simulink model "FOC_physical_2"  (R2024b)
settings: Solver=FixedStepAuto  StartTime=0.0  StopTime=1  FixedStep=1e-6  RelTol=1e-3
undefined symbols (not defined in the file): alpha, DiscIntNeverNeededParam, Down, dspblkCoreblockFVToolHelper, gcbh, GPTRIP1SEL, Ki_current, Ki_q, Ki_s, Ki_speed, Kp_current, Kp_q, Kp_s, Kp_speed, lambda, lamdaM, Ld, Ls, ma, P, Rs, T_max, T_period, TZ1, Up, Vdc
libraries: c2802xlib x7, simulink x7, spsIGBTDiodeLib x6, spsCurrentMeasurementLib x3, eeStairGenerator x2, spsDCVoltageSourceLib x1, spsPermanentMagnetSynchronousMachineLib x1, mcbpositiondecoderlib x1, c281xlib x1, c280xlib x1, spspowerguiLib x1
(part 2 of 2)

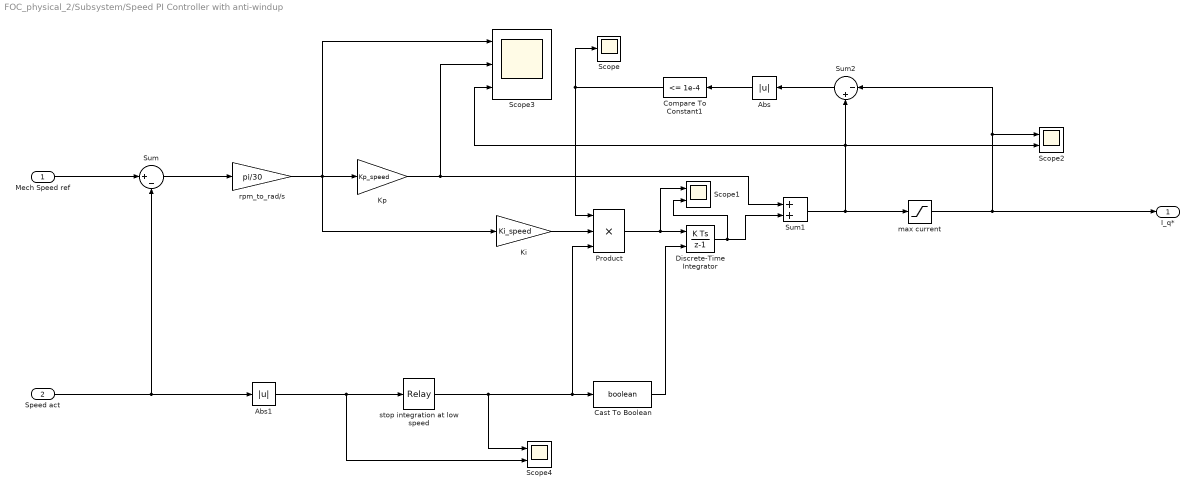
== system FOC_physical_2/Subsystem/Speed PI Controller with anti-windup ==
  Mech Speed ref : Inport
  Speed act : Inport  Port=2
  " max current" : Saturate  UpperLimit=T_max/((3/2)*lamdaM*P)  LowerLimit=0
  Abs : Abs  SaturateOnIntegerOverflow=off
  Abs1 : Abs  SaturateOnIntegerOverflow=off
  Cast To Boolean : DataTypeConversion  OutDataTypeStr=boolean  SaturateOnIntegerOverflow=off  RndMeth=Floor
  Compare To Constant1 : simulink/Logic and Bit Operations/Compare To Constant  relop=<=  const=1e-4  OutDataTypeStr=boolean
  Discrete-Time Integrator : DiscreteIntegrator  ExternalReset=falling  SampleTime=-1  ICPrevOutput=DiscIntNeverNeededParam  ICPrevScaledInput=DiscIntNeverNeededParam
  "Ki " : Gain  Gain=Ki_speed
  Kp : Gain  Gain=Kp_speed
  Product : Product  Inputs=3
  Scope : Scope
  Scope1 : Scope  NumInputPorts=2
  Scope2 : Scope  NumInputPorts=2
  Scope3 : Scope  NumInputPorts=3
  Scope4 : Scope  NumInputPorts=2
  Sum : Sum  Inputs=|+-
  Sum1 : Sum
  Sum2 : Sum  Inputs=|-+
  rpm_to_rad/s : Gain  Gain=pi/30
  stop integration at low speed : Relay  OnSwitchValue=100  OffSwitchValue=-100
  I_q* : Outport
  wires:
  " max current"/1 -> Scope2/1, Sum2/1, I_q*/1
  Sum/1 -> rpm_to_rad/s/1
  rpm_to_rad/s/1 -> Kp/1, Scope3/1, "Ki "/1
  stop integration at low speed/1 -> Cast To Boolean/1, Product/3, Scope4/1
  Abs1/1 -> Scope4/2, stop integration at low speed/1
  Compare To Constant1/1 -> Scope/1, Product/1
  Abs/1 -> Compare To Constant1/1
  Sum2/1 -> Abs/1
  Sum1/1 -> " max current"/1, Sum2/2, Scope3/3, Scope2/2
  Discrete-Time Integrator/1 -> Sum1/2, Scope1/2
  Product/1 -> Discrete-Time Integrator/1, Scope1/1
  "Ki "/1 -> Product/2
  Kp/1 -> Sum1/1, Scope3/2
  Speed act/1 -> Sum/2, Abs1/1
  Mech Speed ref/1 -> Sum/1
  Cast To Boolean/1 -> Discrete-Time Integrator/2

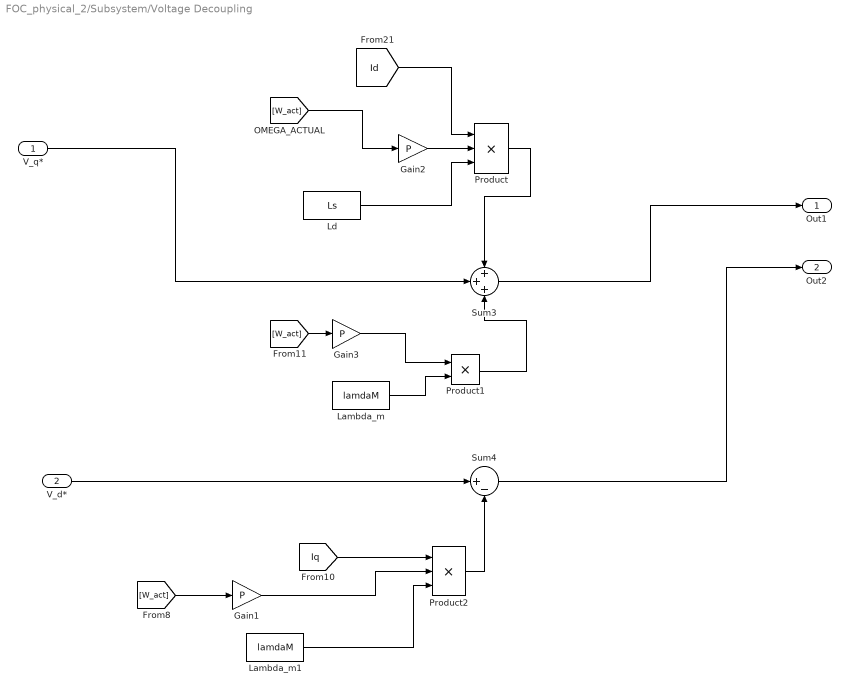
== system FOC_physical_2/Subsystem/Voltage Decoupling  ==
  V_q* : Inport
  V_d* : Inport  Port=2
  Gain1 : Gain  Gain=P
  Gain2 : Gain  Gain=P
  Gain3 : Gain  Gain=P
  Lambda_m : Constant  Value=lamdaM
  Lambda_m1 : Constant  Value=lamdaM
  Ld : Constant  Value=Ls
  Product : Product  Inputs=3
  Product1 : Product
  Product2 : Product  Inputs=3
  Sum3 : Sum  Inputs=+++
  Sum4 : Sum  Inputs=|+-
  Out1 : Outport
  Out2 : Outport  Port=2
  wires:
  [Id] -> Product/1
  V_q*/1 -> Sum3/2
  Gain1/1 -> Product2/2
  Product2/1 -> Sum4/2
  [Iq] -> Product2/1
  Product1/1 -> Sum3/3
  [W_act] -> Gain1/1
  Gain2/1 -> Product/2
  [W_act] -> Gain2/1
  Ld/1 -> Product/3
  [W_act] -> Gain3/1
  Product/1 -> Sum3/1
  Gain3/1 -> Product1/1
  Lambda_m/1 -> Product1/2
  Lambda_m1/1 -> Product2/3
  Sum3/1 -> Out1/1
  V_d*/1 -> Sum4/1
  Sum4/1 -> Out2/1

== system FOC_physical_2/Subsystem/d-current PI controller with anti-windup ==
  Id command : Inport
  Id act : Inport  Port=2
  Discrete-Time Integrator : DiscreteIntegrator  SampleTime=-1  ICPrevOutput=DiscIntNeverNeededParam  ICPrevScaledInput=DiscIntNeverNeededParam
  "Ki " : Gain  Gain=Ki_current
  Kp : Gain  Gain=Kp_current
  Product : Product
  Scope : Scope
  Scope1 : Scope  NumInputPorts=2
  Scope2 : Scope  NumInputPorts=2
  Scope3 : Scope  NumInputPorts=3
  Sum : Sum  Inputs=|+-
  Sum1 : Sum
  V_d* : Outport
  wires:
  Sum1/1 -> V_d*/1, Scope3/3, Scope2/2
  Discrete-Time Integrator/1 -> Sum1/2, Scope1/2
  Product/1 -> Discrete-Time Integrator/1, Scope1/1
  "Ki "/1 -> Product/2
  Kp/1 -> Sum1/1, Scope3/2
  Sum/1 -> Kp/1, Scope3/1, "Ki "/1
  Id act/1 -> Sum/2
  Id command/1 -> Sum/1
  [stop_d_integrator] -> Product/1, Scope/1

== system FOC_physical_2/Subsystem/q-current PI controller with anti-windup ==
  Iq command : Inport
  Iq act : Inport  Port=2
  Discrete-Time Integrator : DiscreteIntegrator  SampleTime=-1  ICPrevOutput=DiscIntNeverNeededParam  ICPrevScaledInput=DiscIntNeverNeededParam
  "Ki " : Gain  Gain=Ki_current
  Kp : Gain  Gain=Kp_current
  Product : Product
  Scope : Scope
  Scope1 : Scope  NumInputPorts=2
  Scope2 : Scope  NumInputPorts=2
  Scope3 : Scope  NumInputPorts=3
  Sum : Sum  Inputs=|+-
  Sum1 : Sum
  V_q* : Outport
  wires:
  Iq command/1 -> Sum/1
  Iq act/1 -> Sum/2
  Sum/1 -> "Ki "/1, Scope3/1, Kp/1
  Kp/1 -> Scope3/2, Sum1/1
  "Ki "/1 -> Product/2
  Product/1 -> Discrete-Time Integrator/1, Scope1/1
  Discrete-Time Integrator/1 -> Scope1/2, Sum1/2
  Sum1/1 -> V_q*/1, Scope2/2, Scope3/3
  [stop_q_integrator] -> Scope/1, Product/1

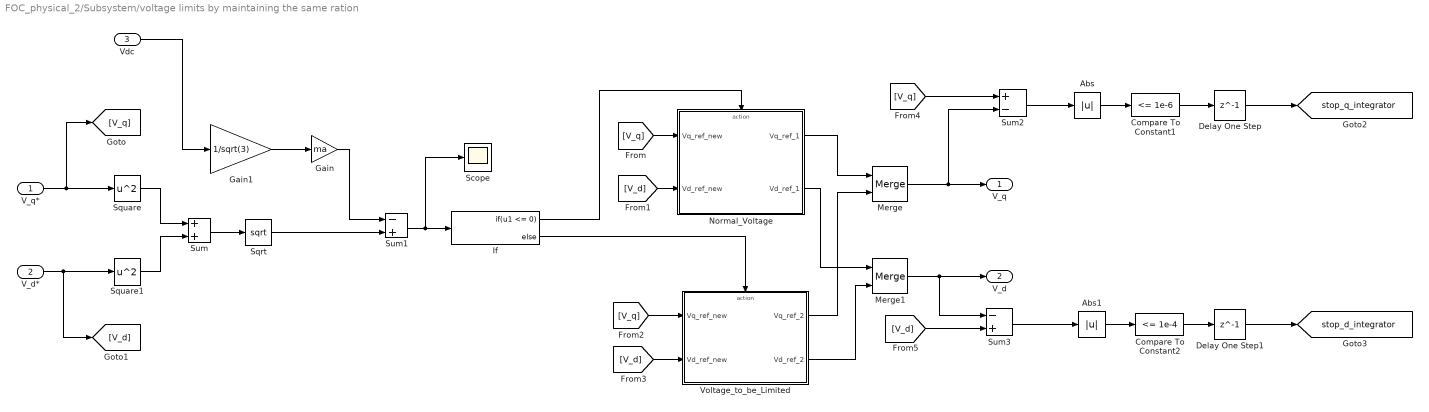
== system FOC_physical_2/Subsystem/voltage limits by maintaining the same ration ==
  V_q* : Inport
  V_d* : Inport  Port=2
  Vdc : Inport  Port=3
  Abs : Abs  SaturateOnIntegerOverflow=off
  Abs1 : Abs  SaturateOnIntegerOverflow=off
  Compare To Constant1 : simulink/Logic and Bit Operations/Compare To Constant  relop=<=  const=1e-6  OutDataTypeStr=boolean
  Compare To Constant2 : simulink/Logic and Bit Operations/Compare To Constant  relop=<=  const=1e-4  OutDataTypeStr=boolean
  Delay One Step : Delay  DelayLength=1
  Delay One Step1 : Delay  DelayLength=1
  Gain : Gain  Gain=ma
  Gain1 : Gain  Gain=1/sqrt(3)
  If : If  IfExpression=u1 <= 0
  Merge : Merge
  Merge1 : Merge
  Normal_Voltage : Subsystem  TreatAsAtomicUnit=on
      settings: RTWSystemCode=Inline  RTWFcnNameOpts=Use subsystem name  RTWFileNameOpts=Use subsystem name
  Scope : Scope
  Sqrt : Sqrt
  Square : Math  Operator=square
  Square1 : Math  Operator=square
  Sum : Sum
  Sum1 : Sum  Inputs=-+
  Sum2 : Sum  Inputs=+-
  Sum3 : Sum  Inputs=-+
  Voltage_to_be_Limited : Subsystem  TreatAsAtomicUnit=on
      settings: RTWSystemCode=Inline  RTWFcnNameOpts=Use subsystem name  RTWFileNameOpts=Use subsystem name
  V_q : Outport
  V_d : Outport  Port=2
  tag scope: stop_d_integrator=global, stop_q_integrator=global
  wires:
  V_q*/1 -> [V_q], Square/1
  V_d*/1 -> [V_d], Square1/1
  Sum/1 -> Sqrt/1
  Square/1 -> Sum/1
  Square1/1 -> Sum/2
  Sqrt/1 -> Sum1/2
  Merge/1 -> Sum2/2, V_q/1
  Gain/1 -> Sum1/1
  Sum1/1 -> Scope/1, If/1
  If/1 -> Normal_Voltage/Action
  [V_q] -> Normal_Voltage/1(Vq_ref_new)
  [V_d] -> Normal_Voltage/2(Vd_ref_new)
  If/2 -> Voltage_to_be_Limited/Action
  Voltage_to_be_Limited/1(Vq_ref_2) -> Merge/2
  Normal_Voltage/1(Vq_ref_1) -> Merge/1
  Voltage_to_be_Limited/2(Vd_ref_2) -> Merge1/2
  Normal_Voltage/2(Vd_ref_1) -> Merge1/1
  [V_q] -> Voltage_to_be_Limited/1(Vq_ref_new)
  [V_d] -> Voltage_to_be_Limited/2(Vd_ref_new)
  [V_q] -> Sum2/1
  Merge1/1 -> Sum3/1, V_d/1
  [V_d] -> Sum3/2
  Delay One Step/1 -> [stop_q_integrator]
  Delay One Step1/1 -> [stop_d_integrator]
  Abs/1 -> Compare To Constant1/1
  Compare To Constant1/1 -> Delay One Step/1
  Sum2/1 -> Abs/1
  Sum3/1 -> Abs1/1
  Abs1/1 -> Compare To Constant2/1
  Compare To Constant2/1 -> Delay One Step1/1
  Vdc/1 -> Gain1/1
  Gain1/1 -> Gain/1

== system FOC_physical_2/Voltage limits/If Action Subsystem ==
  In3 : Inport
  In4 : Inport  Port=2
  Action Port : ActionPort  ActionPortLabel=if(u1 <= 0)
  Cast To Single : DataTypeConversion  OutDataTypeStr=single  SaturateOnIntegerOverflow=off  RndMeth=Floor
  Cast To Single1 : DataTypeConversion  OutDataTypeStr=single  SaturateOnIntegerOverflow=off  RndMeth=Floor
  Out2 : Outport
  Out3 : Outport  Port=2
  wires:
  In3/1 -> Cast To Single/1
  In4/1 -> Cast To Single1/1
  Cast To Single/1 -> Out2/1
  Cast To Single1/1 -> Out3/1

== system FOC_physical_2/Voltage limits/If Action Subsystem1 ==
  In3 : Inport
  In4 : Inport  Port=2
  Action Port : ActionPort  ActionPortLabel=else
  Divide1 : Product  Inputs=*/  OutDataTypeStr=single
  Divide2 : Product  Inputs=/*  OutDataTypeStr=single
  Gain : Gain  Gain=sqrt(3)
  Gain1 : Gain  Gain=325 * .95
  Gain2 : Gain  Gain=325 * .95
  Square : Math  Operator=square  OutDataTypeStr=single
  Square Root : Sqrt  OutDataTypeStr=single  IntermediateResultsDataTypeStr=single
  Square1 : Math  Operator=square  OutDataTypeStr=single
  Sum : Sum  OutDataTypeStr=single  AccumDataTypeStr=single
  Out2 : Outport
  Out3 : Outport  Port=2
  wires:
  Divide1/1 -> Out2/1
  Divide2/1 -> Out3/1
  Square/1 -> Sum/1
  In3/1 -> Gain1/1, Square/1
  Sum/1 -> Square Root/1
  Gain2/1 -> Divide2/2
  Gain/1 -> Divide2/1, Divide1/2
  Gain1/1 -> Divide1/1
  Square1/1 -> Sum/2
  Square Root/1 -> Gain/1
  In4/1 -> Square1/1, Gain2/1

== system FOC_physical_2/SVPWM Technique/Step 1- Determine Vd, Vq, Vref, and angle/Polar form ==
  In1 : Inport
  In2 : Inport  Port=2
  Add : Sum
  Atan2 : Trigonometry  Operator=atan2
  Sqrt : Sqrt
  Square : Math  Operator=square
  Square1 : Math  Operator=square
  V ref : Outport
  angle : Outport  Port=2
  wires:
  In1/1 -> Square/1, Atan2/2
  Add/1 -> Sqrt/1
  Sqrt/1 -> V ref/1
  In2/1 -> Square1/1, Atan2/1
  Atan2/1 -> angle/1
  Square/1 -> Add/1
  Square1/1 -> Add/2

== system FOC_physical_2/SVPWM Technique/Step 1- Determine Vd, Vq, Vref, and angle/Power variant Clark transformation  ==
  Va : Inport
  Vb : Inport  Port=2
  Vc : Inport  Port=3
  Gain : Gain  Gain=0.5
  Gain1 : Gain  Gain=0.5
  Gain2 : Gain  Gain=2/3
  Gain3 : Gain  Gain=sqrt(3)/2
  Gain4 : Gain  Gain=2/3
  Sum : Sum  Inputs=+--
  Sum1 : Sum  Inputs=+-
  V alpha : Outport
  V beta : Outport  Port=2
  wires:
  Gain4/1 -> V beta/1
  Gain2/1 -> V alpha/1
  Vb/1 -> Gain/1, Sum1/1
  Gain/1 -> Sum/2
  Sum1/1 -> Gain3/1
  Gain1/1 -> Sum/3
  Vc/1 -> Gain1/1, Sum1/2
  Sum/1 -> Gain2/1
  Gain3/1 -> Gain4/1
  Va/1 -> Sum/1

== system FOC_physical_2/SVPWM Technique/Step 2- Determine time duration T1, T2, T/angle_d ==
  angle : Inport
  Sector : Inport  Port=2
  Constant3 : Constant
  Gain : Gain  Gain=pi/3
  Subtract4 : Sum  Inputs=-+
  Subtract5 : Sum  Inputs=+-
  angle_d(0 - pi/3) : Outport
  wires:
  Gain/1 -> Subtract4/1
  Subtract5/1 -> Gain/1
  Constant3/1 -> Subtract5/2
  Subtract4/1 -> angle_d(0 - pi/3)/1
  Sector/1 -> Subtract5/1
  angle/1 -> Subtract4/2

== system FOC_physical_2/Subsystem/Inverse Transformation/Inverse Park  ==
  In1 : Inport
  In2 : Inport  Port=2
  In3 : Inport  Port=3
  Cos : Trigonometry  Operator=cos
  Cos1 : Trigonometry  Operator=cos
  Product{,1..3} (4 alike) : Product
  Sin : Trigonometry
  Sin1 : Trigonometry
  Subtract : Sum  Inputs=+-
  Subtract2 : Sum
  Valpha : Outport
  Vbeta : Outport  Port=2
  wires:
  Product3/1 -> Subtract2/1
  In3/1 -> Product2/2, Product1/2
  In1/1 -> Cos/1, [theta], Sin/1
  Subtract/1 -> Valpha/1  "Valpha"
  Product/1 -> Subtract/1
  Subtract2/1 -> Vbeta/1  "Vbeta"
  Product2/1 -> Subtract2/2
  Cos/1 -> Product/1
  Product1/1 -> Subtract/2
  [theta] -> Cos1/1
  In2/1 -> Product/2, Product3/1
  [theta] -> Sin1/1
  Sin/1 -> Product1/1
  Cos1/1 -> Product2/1
  Sin1/1 -> Product3/2

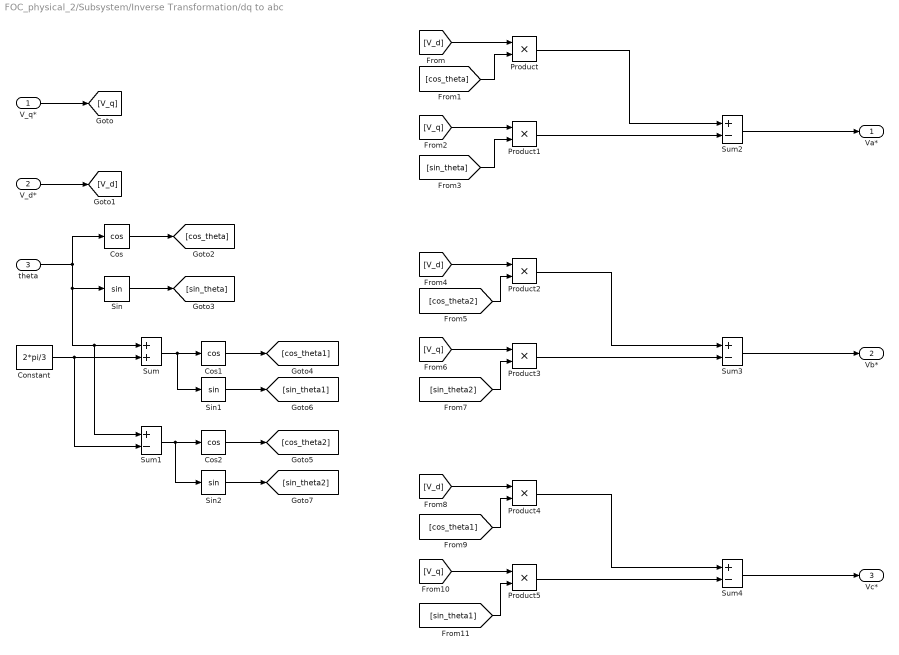
== system FOC_physical_2/Subsystem/Inverse Transformation/dq to abc ==
  V_q* : Inport
  V_d* : Inport  Port=2
  theta : Inport  Port=3
  Constant : Constant  Value=2*pi/3
  Cos : Trigonometry  Operator=cos
  Cos1 : Trigonometry  Operator=cos
  Cos2 : Trigonometry  Operator=cos
  Product{,1..5} (6 alike) : Product
  Sin : Trigonometry
  Sin1 : Trigonometry
  Sin2 : Trigonometry
  Sum : Sum
  Sum{1..4} (4 alike) : Sum  Inputs=+-
  Va* : Outport
  Vb* : Outport  Port=2
  Vc* : Outport  Port=3
  wires:
  [sin_theta1] -> Product5/2
  [V_q] -> Product5/1
  [cos_theta1] -> Product4/2
  [V_d] -> Product4/1
  Product4/1 -> Sum4/1
  Product5/1 -> Sum4/2
  Sum4/1 -> Vc*/1
  [sin_theta2] -> Product3/2
  Sin2/1 -> [sin_theta2]
  Sin1/1 -> [sin_theta1]
  [V_q] -> Product3/1
  [cos_theta2] -> Product2/2
  [V_d] -> Product2/1
  Sum3/1 -> Vb*/1
  Product3/1 -> Sum3/2
  Product2/1 -> Sum3/1
  [sin_theta] -> Product1/2
  [V_q] -> Product1/1
  [cos_theta] -> Product/2
  [V_d] -> Product/1
  Product/1 -> Sum2/1
  Product1/1 -> Sum2/2
  Sum2/1 -> Va*/1
  Cos2/1 -> [cos_theta2]
  Cos1/1 -> [cos_theta1]
  Sum1/1 -> Cos2/1, Sin2/1
  Sum/1 -> Cos1/1, Sin1/1
  Constant/1 -> Sum/2, Sum1/2
  Sin/1 -> [sin_theta]
  Cos/1 -> [cos_theta]
  theta/1 -> Cos/1, Sin/1, Sum1/1, Sum/1
  V_d*/1 -> [V_d]
  V_q*/1 -> [V_q]

== system FOC_physical_2/Subsystem/Inverse Transformation/inverse Clark ==
  In1 : Inport
  In2 : Inport  Port=2
  Add : Sum
  Add1 : Sum
  Constant : Constant  Value=-1/2
  Constant1 : Constant  Value=sqrt(3)/2
  Constant2 : Constant  Value=-1/2
  Constant3 : Constant  Value=-sqrt(3)/2
  Product{,1..3} (4 alike) : Product
  Va : Outport
  Vb : Outport  Port=2
  Vc : Outport  Port=3
  wires:
  In1/1 -> Va/1, Product1/2, Product2/2
  In2/1 -> Product/1, Product3/2
  Add/1 -> Vb/1
  Product3/1 -> Add1/2
  Constant/1 -> Product1/1
  Constant2/1 -> Product2/1
  Product/1 -> Add/2
  Constant1/1 -> Product/2
  Product1/1 -> Add/1
  Product2/1 -> Add1/1
  Add1/1 -> Vc/1
  Constant3/1 -> Product3/1

== system FOC_physical_2/Subsystem/SVPWM1/Subsystem ==
  Valpha : Inport
  Vbeta : Inport  Port=2
  Atan2 : Trigonometry  Operator=atan2
  Display : Display
  Display1 : Display
  Math Function : Math  Operator=square
  Math Function1 : Math  Operator=square
  Scope : Scope
  Sqrt1 : Sqrt
  Sum : Sum  Inputs=|++
  Vref : Outport
  angle : Outport  Port=2
  wires:
  Sum/1 -> Sqrt1/1
  Atan2/1 -> Display1/1, angle/1
  Math Function/1 -> Sum/1
  Sqrt1/1 -> Scope/1, Vref/1, Display/1
  Vbeta/1 -> Math Function1/1, Atan2/1
  Valpha/1 -> Math Function/1, Atan2/2
  Math Function1/1 -> Sum/2

== system FOC_physical_2/Subsystem/SVPWM1/Subsystem1 ==
  Vref : Inport
  angle : Inport  Port=2
  Sector : Inport  Port=3
  Vdc : Inport  Port=4
  Add : Sum  Inputs=--+
  Constant4 : Constant  Value=T_period
  Constant5 : Constant  Value=pi/3
  Divide : Product  Inputs=*/
  Gain : Gain  Gain=(T_period)*sqrt(3)
  Product1 : Product
  Product2 : Product
  Sin : Trigonometry
  Sin1 : Trigonometry
  Subtract3 : Sum  Inputs=+-
  Theta dash : Subsystem
  T1 : Outport
  T2 : Outport  Port=2
  T0 : Outport  Port=3
  wires:
  Theta dash/1(Theta dash) -> Subtract3/2, Sin1/1
  Add/1 -> T0/1
  Product2/1 -> T2/1, Add/2
  Constant4/1 -> Add/3
  Product1/1 -> Add/1, T1/1
  Sin1/1 -> Product2/2
  Sin/1 -> Product1/2
  Gain/1 -> Product1/1, Product2/1
  Subtract3/1 -> Sin/1
  Vdc/1 -> Divide/2
  Vref/1 -> Divide/1
  Divide/1 -> Gain/1
  angle/1 -> Theta dash/2(angle)
  Constant5/1 -> Subtract3/1
  Sector/1 -> Theta dash/1(Sector)

== system FOC_physical_2/Subsystem/SVPWM1/Subsystem2 ==
  T1 : Inport
  T2 : Inport  Port=2
  T0 : Inport  Port=3
  Sector definiton : Inport  Port=4
  Display : Display
  Fcn : Fcn  Expr=(T_period)-(u(3)/2)
  Fcn1 : Fcn  Expr=u(2)+(u(3)/2)
  Fcn2 : Fcn  Expr=u(3)/2
  Fcn3 : Fcn  Expr=u(1)+(u(3)/2)
  MATLAB Function : MATLAB Function  TreatAsAtomicUnit=on
  Mux : Mux  Inputs=3
  TS1 : Outport
  TS3 : Outport  Port=2
  TS5 : Outport  Port=3
  wires:
  Sector definiton/1 -> MATLAB Function/5(S)
  Fcn3/1 -> MATLAB Function/4(g)
  Fcn2/1 -> MATLAB Function/3(w)
  Fcn1/1 -> MATLAB Function/2(v)
  Fcn/1 -> MATLAB Function/1(u)
  Mux/1 -> Fcn2/1, Fcn3/1, Fcn/1, Fcn1/1, Display/1
  T0/1 -> Mux/3
  T2/1 -> Mux/2
  T1/1 -> Mux/1
  MATLAB Function/2(TS3) -> TS3/1
  MATLAB Function/3(TS5) -> TS5/1
  MATLAB Function/1(TS1) -> TS1/1

== system FOC_physical_2/Subsystem/SVPWM1/Subsystem3 ==
  TS1 : Inport
  TS3 : Inport  Port=2
  TS5 : Inport  Port=3
  Carrier : Inport  Port=4
  Relational Operator : RelationalOperator  OutDataTypeStr=boolean  RndMeth=Simplest  InputSameDT=off
  Relational Operator1 : RelationalOperator  OutDataTypeStr=boolean  RndMeth=Simplest  InputSameDT=off
  Relational Operator2 : RelationalOperator  OutDataTypeStr=boolean  RndMeth=Simplest  InputSameDT=off
  Scope : Scope  NumInputPorts=3
  Pwm1 : Outport
  PWM3 : Outport  Port=2
  PWM5 : Outport  Port=3
  wires:
  Relational Operator2/1 -> PWM5/1
  Relational Operator1/1 -> PWM3/1
  Relational Operator/1 -> Pwm1/1, Scope/3
  Carrier/1 -> Relational Operator2/2, Relational Operator1/2, Relational Operator/2, Scope/2
  TS5/1 -> Relational Operator2/1
  TS3/1 -> Relational Operator1/1
  TS1/1 -> Relational Operator/1, Scope/1

== system FOC_physical_2/Subsystem/SVPWM1/Subsystem4 ==
  TS1 : Inport
  TS3 : Inport  Port=2
  TS5 : Inport  Port=3
  NOT : Logic  Operator=NOT  IconShape=distinctive  AllPortsSameDT=off  OutDataTypeStr=boolean
  NOT1 : Logic  Operator=NOT  IconShape=distinctive  AllPortsSameDT=off  OutDataTypeStr=boolean
  NOT2 : Logic  Operator=NOT  IconShape=distinctive  AllPortsSameDT=off  OutDataTypeStr=boolean
  S1 : Outport
  S2 : Outport  Port=2
  S3 : Outport  Port=3
  S4 : Outport  Port=4
  S5 : Outport  Port=5
  S6 : Outport  Port=6
  wires:
  TS1/1 -> NOT/1, S1/1
  NOT/1 -> S4/1
  TS3/1 -> NOT1/1, S3/1
  NOT1/1 -> S6/1
  TS5/1 -> S5/1, NOT2/1
  NOT2/1 -> S2/1

== system FOC_physical_2/Subsystem/SVPWM1/Valpha and Vbeta Clark Trans ==
  Va : Inport
  Vb : Inport  Port=2
  Vc : Inport  Port=3
  Add : Sum  Inputs=+++
  Add1 : Sum  Inputs=+-
  Gain : Gain  Gain=2/3
  Gain1 : Gain  Gain=-1/2
  Gain2 : Gain  Gain=-1/2
  Gain3 : Gain  Gain=2/3
  Gain5 : Gain  Gain=sqrt(3)/2
  Valpha : Outport
  Vbeta : Outport  Port=2
  wires:
  Gain5/1 -> Gain3/1
  Vc/1 -> Gain2/1, Add1/2
  Vb/1 -> Gain1/1, Add1/1
  Gain3/1 -> Vbeta/1
  Gain/1 -> Valpha/1
  Add/1 -> Gain/1
  Gain2/1 -> Add/3
  Add1/1 -> Gain5/1
  Va/1 -> Add/1
  Gain1/1 -> Add/2

== system FOC_physical_2/Subsystem/voltage limits by maintaining the same ration/Normal_Voltage ==
  Vq_ref_new : Inport
  Vd_ref_new : Inport  Port=2
  Action Port : ActionPort  ActionPortLabel=if(u1 <= 0)
  Data Type Conversion : DataTypeConversion  OutDataTypeStr=single  SaturateOnIntegerOverflow=off  RndMeth=Floor
  Data Type Conversion1 : DataTypeConversion  OutDataTypeStr=single  SaturateOnIntegerOverflow=off  RndMeth=Floor
  Vq_ref_1 : Outport
  Vd_ref_1 : Outport  Port=2
  wires:
  Vq_ref_new/1 -> Data Type Conversion/1
  Vd_ref_new/1 -> Data Type Conversion1/1
  Data Type Conversion/1 -> Vq_ref_1/1
  Data Type Conversion1/1 -> Vd_ref_1/1

== system FOC_physical_2/Subsystem/voltage limits by maintaining the same ration/Voltage_to_be_Limited ==
  Vq_ref_new : Inport
  Vd_ref_new : Inport  Port=2
  Action Port : ActionPort  ActionPortLabel=else
  Divide1 : Product  Inputs=*/  OutDataTypeStr=single
  Divide2 : Product  Inputs=/*  OutDataTypeStr=single
  Gain : Gain  Gain=sqrt(3)
  Gain1 : Gain  Gain=Vdc * ma
  Gain2 : Gain  Gain=Vdc * ma
  Square : Math  Operator=square  OutDataTypeStr=single
  Square Root : Sqrt  OutDataTypeStr=single  IntermediateResultsDataTypeStr=single
  Square1 : Math  Operator=square  OutDataTypeStr=single
  Sum : Sum  OutDataTypeStr=single  AccumDataTypeStr=single
  Vq_ref_2 : Outport
  Vd_ref_2 : Outport  Port=2
  wires:
  Vq_ref_new/1 -> Gain1/1, Square/1
  Sum/1 -> Square Root/1
  Vd_ref_new/1 -> Square1/1, Gain2/1
  Square1/1 -> Sum/2
  Square/1 -> Sum/1
  Divide1/1 -> Vq_ref_2/1
  Square Root/1 -> Gain/1
  Divide2/1 -> Vd_ref_2/1
  Gain/1 -> Divide2/1, Divide1/2
  Gain1/1 -> Divide1/1
  Gain2/1 -> Divide2/2

== system FOC_physical_2/Subsystem/SVPWM1/Subsystem1/Theta dash ==
  Sector : Inport
  angle : Inport  Port=2
  Constant : Constant
  Display : Display
  Gain : Gain  Gain=(pi/3)
  Subtract : Sum  Inputs=-+
  Subtract1 : Sum  Inputs=-+
  Theta dash : Outport
  wires:
  Subtract/1 -> Theta dash/1, Display/1
  Subtract1/1 -> Gain/1
  Sector/1 -> Subtract1/2
  Constant/1 -> Subtract1/1
  Gain/1 -> Subtract/1
  angle/1 -> Subtract/2

== matlab function FOC_physical_2/SVPWM Technique/Sector Detector ==
  data: u input; S output
function S = fcn(u)

  u= 180/(pi)*u ; % rad to degree
  
if (u>=0)&&(u<60)
  u = 1  ; 
elseif (u>=60)&&(u<120)
  u = 2  ;  
elseif (u>=120)&&(u<180)
  u = 3  ;  
elseif (u>=-180)&&(u<-120)
  u = 4  ;
elseif (u>=-120)&&(u<-60)
  u = 5  ;
elseif (u>=-60)&&(u<0)
  u = 6  ;
else
  u=0 ; 
end

S = u;

== matlab function FOC_physical_2/SVPWM Technique/Step 3- Determine the switching time of each transistor (S1 to S6) /Sector detection1 ==
  data: s input; u input; Ts1 output; Ts3 output; v input; w input; g input; Ts5 output
function [Ts1,Ts3,Ts5] = fcn(s,u,v,w,g)

switch s 
  
 case 1 
  Ts1 = u ; 
  Ts3 = v ;
  Ts5 = w ;
 case 2 
  Ts1 = g ; 
  Ts3 = u ; 
  Ts5 = w ;
 case 3 
  Ts1 = w ;
  Ts3 = u ; 
  Ts5 = v ; 
 case 4 
  Ts1 = w ;
  Ts3 = g ; 
  Ts5 = u ;
 case 5 
  Ts1 = v ;
  Ts3 = w ; 
  Ts5 = u ;
 case 6 
  Ts1 = u ;
  Ts3 = w ; 
  Ts5 = g ;
 otherwise 
 Ts1 = 0 ; 
 Ts3 = 0 ;
 Ts5 = 0 ;
 end 

end

== matlab function FOC_physical_2/Subsystem1/MATLAB Function ==
  data: theta input; speed_rad_s output; Ts input
function speed_rad_s = calculate_speed(theta, Ts)
    % persistent variable remembers the angle from the previous time step
    persistent theta_prev;
    if isempty(theta_prev)
        theta_prev = 0;
    end

    % Calculate the raw delta
    delta_theta = theta - theta_prev;

    % UNWRAP LOGIC: Fix the jump from 2*pi to 0 (and vice versa)
    if delta_theta < -pi
        delta_theta = delta_theta + 2*pi;
    elseif delta_theta > pi
        delta_theta = delta_theta - 2*pi;
    end

    % Calculate speed and update previous value
    speed_rad_s = delta_theta / Ts;
    theta_prev = theta;
end

== matlab function FOC_physical_2/Subsystem/SVPWM1/Sector detection ==
  data: u input; S output
function S = fcn(u)

u = (180/pi)* u;

if(u < 60 && u >= 0)
    u = 1;
elseif(u < 120 && u >= 60)
    u = 2;
elseif(u < 180 && u >= 120)
    u = 3;
elseif(u < -120 && u >= -180)
u = 4;
elseif(u < -60 && u >= -120)
u = 5;
elseif(u < 0 && u >= -60)
u = 6;
else
    u = 0;
end
S = u;

== matlab function FOC_physical_2/Subsystem/SVPWM1/Subsystem2/MATLAB Function ==
  data: TS1 output; u input; TS3 output; TS5 output; v input; w input; g input; S input
function [TS1, TS3,TS5] = fcn(u, v, w, g,S)

switch S
    case 1
        TS1 = u;
        TS3 = v;
        TS5 = w;
    case 2
        TS1 = g;
        TS3 = u;
        TS5 = w;
    case 3
        TS1 = w;
        TS3 = u;
        TS5 = v;
    case 4
        TS1 = w;
        TS3 = g;
        TS5 = u;
    case 5
        TS1 = v;
        TS3 = w;
        TS5 = u;
    case 6
        TS1 = u;
        TS3 = w;
        TS5 = g;
    otherwise
      TS1=0;  
      TS3=0;  
      TS5=0; 
end
end
